simulink model "Arduino_assignment"  (R2020b)
settings: Solver=FixedStepDiscrete  StartTime=0.0  StopTime=10.0  FixedStep=1e-4  RelTol=1e-3  EnableMultiTasking=on
libraries: arduinolib x3
settings Model: SILPILModeSetting=veronly  ExtModeTrigDuration=2  Creator=salvo  LastModifiedBy=salvo
settings OptimizationCC: EnhancedBackFolding=on  PassReuseOutputArgsAs=Individual arguments  ZeroExternalMemoryAtStartup=off  ZeroInternalMemoryAtStartup=off  MaxStackSize=64  OptimizeBlockOrder=speed  DifferentSizesBufferReuse=on  OptimizationCustomize=off  EfficientTunableParamExpr=on
settings DebuggingCC: ParameterTunabilityLossMsg=error
settings HardwareCC: ProdBitPerInt=16  ProdBitPerPointer=16  ProdBitPerSizeT=16  ProdBitPerPtrDiffT=16  ProdLargestAtomicFloat=None  ProdWordSize=8  ProdHWDeviceType=Atmel->AVR
settings SFSimCC: MATLABDynamicMemAlloc=off
settings RTWCC: Description=Embedded Coder  SystemTargetFile=ert.tlc  HardwareBoard=Arduino Uno  TemplateMakefile=ert_default_tmf  Toolchain=Arduino AVR  BuildConfiguration=Faster Runs
settings CodeAppCC: ForceParamTrailComments=on  IgnoreCustomStorageClasses=off  OperatorAnnotations=on  SimulinkDataObjDesc=on  SFDataObjDesc=on  InsertBlockDesc=on
settings ERTTargetCC: SupportContinuousTime=on  SupportVariableSizeSignals=on  ExtModeStaticAllocSize=250

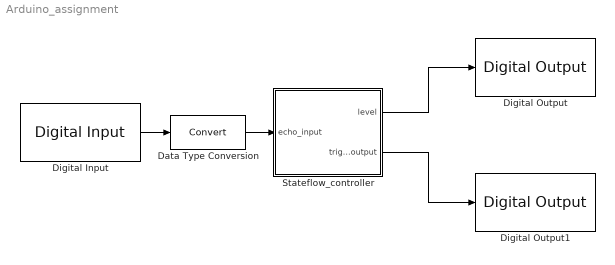
== system Arduino_assignment ==
  Data Type Conversion : DataTypeConversion
  Digital Input : arduinolib/Digital Input  pinNumber=11  mode=Default  Direction=input  SampleTime=0.0001  blockPlatform=arduino
  Digital Output : arduinolib/Digital Output  pinNumber=13  Direction=output  blockPlatform=arduino
  Digital Output1 : arduinolib/Digital Output  pinNumber=12  Direction=output  blockPlatform=arduino
  Stateflow_controller : Stateflow chart  TreatAsAtomicUnit=on
  wires:
  Stateflow_controller/1(level) -> Digital Output/1
  Stateflow_controller/2(trigger_output) -> Digital Output1/1
  Digital Input/1 -> Data Type Conversion/1
  Data Type Conversion/1 -> Stateflow_controller/1(echo_input)

== stateflow chart Arduino_assignment/Stateflow_controller ==
  state TRIGGER [parallel]
    settings: executionOrder=1
    state TRIGGER_ON
      en:
      trigger_output=1;
    state TRIGGER_OFF
      en:
      trigger_output=0;
    (default) -> TRIGGER_ON
    TRIGGER_OFF -> TRIGGER_ON : after(60, msec)
    TRIGGER_ON -> TRIGGER_OFF : after(100, usec)
  state LOGIC_OPERATOR [parallel]
    settings: executionOrder=2
    state INITIAL_STATE
      en:
      dist_v=[0 0 0 0]';
      i=1;
      counter=0;
      mean=0;
    state COUNTER
      en,du:
      counter= counter + 100;
    state ERROR
      en:
      up=0.5;
      down=0.5;
    state SAVE_MEASURE
      en:
      dist_v(i)=counter;
    state MEAN
      en:
      mean=(dist_v(1)+dist_v(2)+dist_v(3)+dist_v(4))/232;
      dist_v(1)=dist_v(2);
      dist_v(2)=dist_v(3);
      dist_v(3)=dist_v(4);
      i=4;
    state OUT_RANGE
      en:
      up=0.25;
      down=0.25;
    state IN_RANGE
      en:
      up=(mean*0.001);
      down=(0.1-up);
    (default) -> INITIAL_STATE
    (junction 45) -> INITIAL_STATE
    ERROR -> (junction 45)
    INITIAL_STATE -> (junction 48) [order 2] : after(0.0601, sec)
    (junction 48) -> ERROR
    INITIAL_STATE -> COUNTER [order 1] : [echo_input==1]
    (junction 32) -> COUNTER
    (junction 31) -> (junction 32)
    SAVE_MEASURE -> COUNTER [order 2] : [echo_input==1]{counter=0, i=i+1}
    COUNTER -> SAVE_MEASURE : [echo_input == 0]
    SAVE_MEASURE -> ERROR [order 3] : after(0.0601, sec)
    SAVE_MEASURE -> MEAN [order 1] : [i==4]
    (junction 41) -> ERROR
    MEAN -> IN_RANGE [order 1] : [mean>=10 && mean<=100]
    MEAN -> OUT_RANGE [order 2]
    OUT_RANGE -> (junction 31) [order 1] : [echo_input==1]{counter=0}
    OUT_RANGE -> (junction 36) [order 2] : after(0.0601, sec)
    IN_RANGE -> (junction 31) [order 1] : [echo_input==1]{counter=0}
    IN_RANGE -> (junction 38) [order 2] : after(0.0601, sec)
    (junction 38) -> (junction 41)
    (junction 36) -> (junction 38)
  state LED [parallel]
    settings: executionOrder=3
    state OFF
      en:
      level=0;
    state ON
      en:
      level=1;
    (default) -> OFF
    ON -> OFF : after(up, sec)[down]
    OFF -> ON : after(down, sec)
  data: echo_input input uint8; level output uint8; trigger_output output uint8; counter local uint16; mean local double; i local uint8; dist_v local double; up local double =2; down local double =2
